simulink model "Matlabproject1"  (R2013a)
settings: Solver=ode45  StartTime=0.0  StopTime=10.0  RelTol=1e-3
undefined symbols (not defined in the file): KePhi, T_L, Va
settings Model: Creator=Rajanish kumar  LastModifiedBy=Rajanish kumar

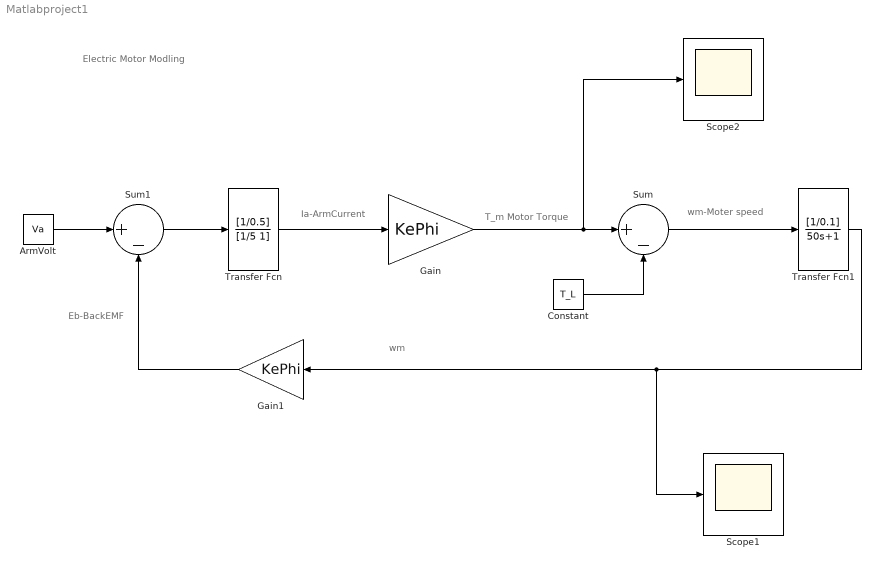
== system Matlabproject1 ==
  note: Electric Motor Modling
  note: wm-Moter speed
  note: T_m Motor Torque
  note: Eb-BackEMF
  note: wm
  note: Ia-ArmCurrent
  ArmVolt : Constant  Value=Va
  Constant : Constant  Value=T_L
  Gain : Gain  Gain=KePhi
  Gain1 : Gain  Gain=KePhi
  Scope1 : Scope
      settings: TimeRange=10  SaveName=wm  Decimation=2
  Scope2 : Scope
      settings: TimeRange=10  YMin=0  YMax=400  SaveName=T_m  Decimation=2
  Sum : Sum  Inputs=|+-
  Sum1 : Sum  Inputs=|+-
  Transfer Fcn : TransferFcn  Numerator=[1/0.5]  Denominator=[1/5 1]
  Transfer Fcn1 : TransferFcn  Numerator=[1/0.1]  Denominator=[50 1]
  wires:
  ArmVolt/1 -> Sum1/1
  Gain1/1 -> Sum1/2
  Sum1/1 -> Transfer Fcn/1
  Transfer Fcn/1 -> Gain/1
  Gain/1 -> Scope2/1, Sum/1
  Constant/1 -> Sum/2
  Sum/1 -> Transfer Fcn1/1
  Transfer Fcn1/1 -> Scope1/1, Gain1/1
